simulink model "SA_50_SIMPLE_MOSFET"  (R2021a)
settings: Solver=VariableStepAuto  StartTime=0.0  StopTime=simTime  RelTol=1e-3
undefined symbols (not defined in the file or in its folder): Iend, Inom, Ion, linearMPC, Lithium, modelSelection, nomAirP, nomFuelP, nomH20comp, nomH2comp, nomO2comp, powerProfile, sigbuilder_block, slow_linearMPC, v_0A, v_1A, Vend, Vnom
libraries: spsCurrentMeasurementLib x3, spsControlledCurrentSourceLib x2, spspowerguiLib x1, spsBatteryLib x1, spsControlledVoltageSourceLib x1, spsDiodeLib x1, spsFirstOrderFilterLib x1, spsFuelCellStackLib x1, spsSeriesRLCBranchLib x1
settings Model: Creator=leonardopalacios  LastModifiedBy=leonardopalacios
settings SolverCC: ZeroCrossAlgorithm=Adaptive
settings DebuggingCC: MaskedZcDiagnostic=none  IgnoredZcDiagnostic=none

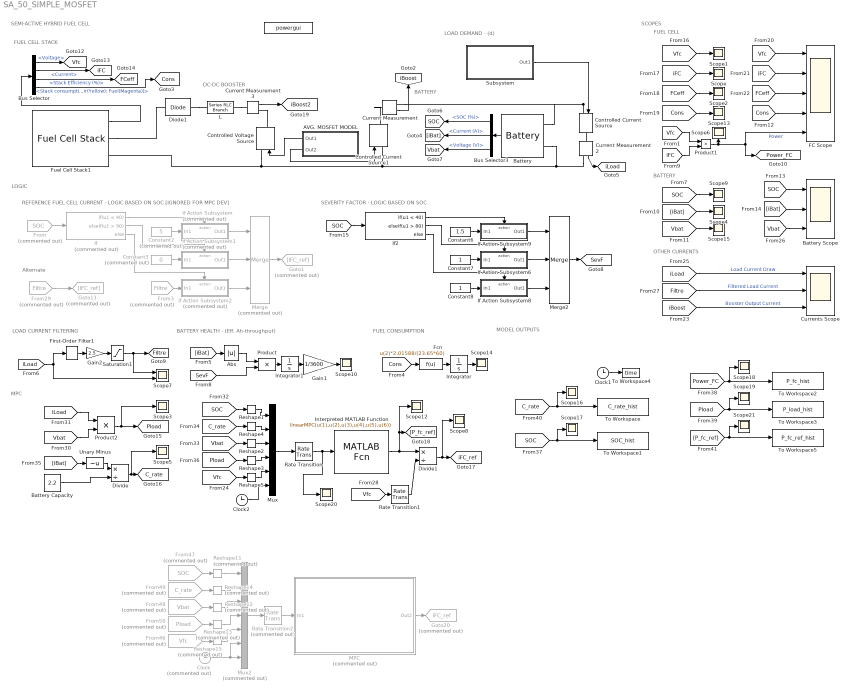
== system SA_50_SIMPLE_MOSFET ==
  note: MODEL OUTPUTS
  note: REFERENCE FUEL CELL CURRENT - LOGIC BASED ON SOC [IGNORED FOR MPC DEV]
  note: BATTERY HEALTH - (Eff. Ah-throughput)
  note: FUEL CELL STACK
  note: LOAD DEMAND - (d)
  note: OTHER CURRENTS
  note: FUEL CONSUMPTION
  note: LOGIC
  note: DC-DC BOOSTER
  note: SEVERITY FACTOR - LOGIC BASED ON SOC
  note: FUEL CELL
  note: BATTERY
  note: BATTERY
  note: LOAD CURRENT FILTERING
  note: SEMI-ACTIVE HYBRID FUEL CELL
  note: SCOPES
  note: MPC
  note: Alternate
  " " : spspowerguiLib/powergui  Priority=1  SimulationMode=Continuous  SampleTime=50e-6  frequency=60  Iterations=50  frequencyindice=0  Pbase=100e6  ErrMax=1e-4  UnitsV=kV  UnitsW=MW  buscounter=0  FunctionMessages=off  echomessages=off  EnableUseOfTLC=off  CurrentSourceSwitches=off  DisableSnubberDevices=off  DisableRonSwitches=off  DisableVfSwitches=off  DisplayEquations=off  AutomaticDiscreteSolvers=off  SolverType=Tustin/Backward Euler (TBE)  Interpol=off  ExternalGateDelay=off  methode=off  Ts=10  x0status=blocks  SPID=off  SwTol=0  HookPort=off  NonlinearTolerance=1e-4  nMaxIteration=100  ContinueOnMaxIteration=off  RestoreLinks=warning  ResistiveCurrentMeasurement=off  Frange=[0:2:500]  Ylog=off  Xlog=on  ShowGrid=off  save=off  variable=ZData  structure=0  ZoomFFT=off  StartTime=0.0  cycles=1  DisplayStyle=1  fundamental=60  FreqAxis=off  MaxFrequency=1000  frequencyindicesteady=1  RmsSteady=1  display=off
  AVG. MOSFET MODEL : Subsystem
  Abs : Abs
  Battery : spsBatteryLib/Battery  BatType=Lithium-Ion  ShowTempParam=off  ThermalPreset=no  ShowAgeParam=off  NomV=bat_nom_V  NomQ=capacity  SOC=SoC_init  Batt_Tr=bat_tau  PresetModel=on  MaxQ=2.2  MinV=30  FullV=46.5595  Dis_rate=0.95652  R=0.18182  Normal_OP=1.9896  expZone="[43.2154     0.108087]"  current=[6.5 13 32.5]  Units=Time  Tci=20  NomT=25  T2=0  MaxQ2=2.208  FullV2=3.45  Normal_OP2=2.8  expZone2="[3.22        0.23]"  Rca=0.6  ti=1000  Dp=0  Neq0=0  Tsim=1e6  Ta1=25  Qeol=5.4*0.9  Reol=0.013333*1.2  Char_age=[2.3478, 3]  Dis_age=[2.3478, 10]  N1=1500  N2=10500  N3=1000  N4=1400  Ta2=45  N5=950
  Battery Capacity : Constant  Value=2.2
  "Battery Scope " : Scope  NumInputPorts=3
  Bus Selector : BusSelector  OutputSignals=Voltage,Current,Stack Efficiency (%),Stack consumption (Standard lpm) [Air(Yellow); Fuel(Magenta)]
  Bus Selector3 : BusSelector  OutputSignals=SOC (%),Current (A),Voltage (V)
  Clock : Clock  Commented=on
  Clock1 : Clock
  Clock2 : Clock
  Constant2 : Constant  Commented=on  Value=5
  Constant3 : Constant  Commented=on  Value=0
  Constant6 : Constant  Value=1.5
  Constant7 : Constant
  Constant8 : Constant
  Controlled Current Source : spsControlledCurrentSourceLib/Controlled Current Source  Initialize=off  Source_Type=DC  Amplitude=0  Phase=0  Frequency=0  Measurements=Current
  Controlled Current Source1 : spsControlledCurrentSourceLib/Controlled Current Source  Initialize=on  Source_Type=DC  Amplitude=0  Phase=0  Frequency=0  Measurements=Current
  Controlled Voltage Source : spsControlledVoltageSourceLib/Controlled Voltage Source  Initialize=on  Source_Type=DC  Amplitude=32.5  Phase=0  Frequency=0  Measurements=None
  Current Measurement : spsCurrentMeasurementLib/Current Measurement  PhasorSimulation=off  OutputType=Complex  PSBequivalent=0
  Current Measurement2 : spsCurrentMeasurementLib/Current Measurement  PhasorSimulation=off  OutputType=Complex  PSBequivalent=0
  Current Measurement3 : spsCurrentMeasurementLib/Current Measurement  PhasorSimulation=off  OutputType=Complex  PSBequivalent=0
  "Currents Scope " : Scope  NumInputPorts=3
  Diode1 : spsDiodeLib/Diode  Ron=0.001  Lon=0  Vf=0.8  IC=0  UseSnubber=off  Rs=500  Cs=250e-9  Measurements=off
  Divide : Product  Inputs=*/
  Divide1 : Product  Inputs=*/
  FC Scope : Scope  NumInputPorts=5
  Fcn : Fcn  Expr=u(2)*2.01588/(23.65*60)
  First-Order Filter1 : spsFirstOrderFilterLib/First-Order Filter  FilterType=Lowpass  Tc=5  Ts=0  Initialize=on  Vac_Init=[0, 0, 60]  Vdc_Init=1.1  PlotResponse=off  FreqRange="[0,  200,  1]"
  From : From  Commented=on  GotoTag=SOC
  From29 : From  Commented=on  GotoTag=Filtre
  From3 : From  Commented=on  GotoTag=Filtre
  From46 : From  Commented=on  GotoTag=Vfc  TagVisibility=global
  From47 : From  Commented=on  GotoTag=SOC  TagVisibility=global
  From48 : From  Commented=on  GotoTag=Vbat  TagVisibility=global
  From49 : From  Commented=on  GotoTag=C_rate  TagVisibility=global
  From50 : From  Commented=on  GotoTag=Pload  TagVisibility=global
  Fuel Cell Stack1 : spsFuelCellStackLib/Fuel Cell Stack  PresetModel=No (User-Defined)  FcType=0  Detailed=Detailed  Eoc=[v_0A, v_1A]  NomVI=[Inom, Vnom]  EndVI=[Iend, Vend]  Nc=nCells  n=stackEff  TOp=opTemp  AirFr=nomAir  SuppPress=[nomFuelP, nomAirP]  Comp=[nomH2comp, nomO2comp, nomH20comp]  SignX=off  SignY=off  FlowRateH2=off  FlowRateAir=off  SystemTemp=off  SystemPH2=off  SystemPAir=off  FCDyn=off  FC_tau=1  Peak_O2=80  V_Under=10
      settings: SourceProductBaseCode=PS
  Gain1 : Gain  Gain=1/3600
  Gain2 : Gain  Gain=2.5
  Goto1 : Goto  Commented=on  GotoTag=iFC_ref
  Goto11 : Goto  Commented=on  GotoTag=iFC_ref
  Goto20 : Goto  Commented=on  GotoTag=iFC_ref  TagVisibility=global
  If : If  Commented=on  IfExpression=u1 < 40  ElseIfExpressions=u1 > 90
  If Action Subsystem : Subsystem  Commented=on  TreatAsAtomicUnit=on
  If Action Subsystem1 : Subsystem  Commented=on  TreatAsAtomicUnit=on
  If Action Subsystem2 : Subsystem  Commented=on  TreatAsAtomicUnit=on
  If Action Subsystem6 : Subsystem  TreatAsAtomicUnit=on
  If Action Subsystem8 : Subsystem  TreatAsAtomicUnit=on
  If Action Subsystem9 : Subsystem  TreatAsAtomicUnit=on
  If2 : If  IfExpression=u1 < 40  ElseIfExpressions=u1 > 80
  Integrator : Integrator
  Integrator1 : Integrator
  Interpreted MATLAB Function : MATLABFcn  MATLABFcn=linearMPC(u(1),u(2),u(3),u(4),u(5),u(6))
  L : spsSeriesRLCBranchLib/Series RLC Branch  LConnTagsString=__new0  RConnTagsString=__new0  BranchType=L  Resistance=1  Inductance=100e-3  SetiL0=off  InitialCurrent=0  Capacitance=1e-6  Setx0=off  InitialVoltage=0  Measurements=None
  MPC : Subsystem  Commented=on
  Merge : Merge  Commented=on  Inputs=3
  Merge2 : Merge  Inputs=3
  Mux : Mux  Inputs=6
  Mux2 : Mux  Commented=on  Inputs=7
  Product : Product
  Product1 : Product
  Product2 : Product
  Rate Transition : RateTransition  OutPortSampleTime=Ts
  Rate Transition1 : RateTransition  OutPortSampleTime=Ts
  Rate Transition2 : RateTransition  Commented=on  OutPortSampleTime=Ts
  Reshape{1..5} (5 alike) : Reshape  OutputDimensionality=Customize  OutputDimensions=1
  Reshape{11..15} (5 alike) : Reshape  Commented=on  OutputDimensionality=Customize  OutputDimensions=1
  Saturation1 : Saturate  UpperLimit=5  LowerLimit=0
  Scope{,1..6,8..10,12..21} (20 alike) : Scope
  Scope7 : Scope  NumInputPorts=2
  Subsystem : Subsystem
  To Workspace : ToWorkspace  VariableName=C_rate_hist  SaveFormat=Timeseries  SampleTime=-1
  To Workspace1 : ToWorkspace  VariableName=SOC_hist  SaveFormat=Timeseries  SampleTime=-1
  To Workspace2 : ToWorkspace  VariableName=P_fc_hist  SaveFormat=Timeseries  SampleTime=-1
  To Workspace3 : ToWorkspace  VariableName=P_load_hist  SaveFormat=Timeseries  SampleTime=-1
  To Workspace4 : ToWorkspace  VariableName=time  SaveFormat=Timeseries  SampleTime=-1
  To Workspace5 : ToWorkspace  VariableName=P_fc_ref_hist  SaveFormat=Timeseries  SampleTime=-1
  Unary Minus : UnaryMinus
  tag scope: C_rate=global, Cons=global, FCeff=global, Filtre=global, Pload=global, Power_FC=global, SOC=global, SevF=global, Vbat=global, Vfc=global, iBoost2=global, iBoost=global, iFC=global, iFC_ref=global, iLoad=global
  wires:
  Battery/1 -> Bus Selector3/1
  [SevF] -> Product/2
  Product/1 -> Integrator1/1
  [Vfc] -> FC Scope/1
  [Vfc] -> Product1/1
  [iBat] -> Unary Minus/1
  Current Measurement2/1 -> [iLoad]
  [Vbat] -> Reshape2/1
  Reshape2/1 -> Mux/3
  First-Order Filter1/1 -> Gain2/1
  Product1/1 -> FC Scope/5, [Power_FC], Scope6/1  "Power"
  [iLoad] -> Product2/1
  [Pload] -> Scope19/1, To Workspace3/1
  Constant3/1 -> If Action Subsystem1/1(In1)
  [FCeff] -> FC Scope/3
  Reshape4/1 -> Mux/2
  [Vbat] -> "Battery Scope "/3
  Clock1/1 -> To Workspace4/1
  Bus Selector/1 -> [Vfc]  "<Voltage>"
  [P_fc_ref] -> Scope21/1, To Workspace5/1
  Reshape3/1 -> Mux/4
  Reshape5/1 -> Mux/5
  Bus Selector/2 -> [iFC]  "<Current>"
  Current Measurement/1 -> [iBoost]
  Mux/1 -> Rate Transition/1
  Gain2/1 -> Saturation1/1
  [SOC] -> Scope17/1, To Workspace1/1
  Bus Selector3/3 -> [Vbat]  "<Voltage (V)>"
  [Cons] -> Fcn/1
  If Action Subsystem9/1(Out1) -> Merge2/1
  If Action Subsystem2/1(Out1) -> Merge/3
  Constant8/1 -> If Action Subsystem8/1(In1)
  If/1 -> If Action Subsystem/Action
  Rate Transition1/1 -> Divide1/2
  If2/2 -> If Action Subsystem6/Action
  If/2 -> If Action Subsystem1/Action
  Integrator/1 -> Scope14/1
  Fcn/1 -> Integrator/1
  Bus Selector/4 -> [Cons]  "<Stack consumption (Standard lpm) [Air(Yellow); Fuel(Magenta)]>"
  [SOC] -> Reshape1/1
  If Action Subsystem/1(Out1) -> Merge/1
  Fuel Cell Stack1/1 -> Bus Selector/1
  Battery Capacity/1 -> Divide/2
  [iBat] -> Abs/1
  Bus Selector/3 -> [FCeff]  "<Stack Efficiency (%)>"
  [iBat] -> "Battery Scope "/2
  [iBoost] -> "Currents Scope "/3  "Booster Output Current"
  Abs/1 -> Product/1
  Merge/1 -> Goto1/1
  From29/1 -> Goto11/1
  [Cons] -> FC Scope/4
  If/3 -> If Action Subsystem2/Action
  Divide/1 -> Scope5/1, [C_rate]
  Saturation1/1 -> [Filtre], Scope7/1
  [iLoad] -> "Currents Scope "/1  "Load Current Draw"
  Bus Selector3/1 -> [SOC]  "<SOC (%)>"
  Constant2/1 -> If Action Subsystem/1(In1)
  [C_rate] -> Reshape4/1
  [Filtre] -> "Currents Scope "/2  "Filtered Load Current"
  Divide1/1 -> Scope8/1, [iFC_ref]
  [Vbat] -> Product2/2
  From/1 -> If/1
  Product2/1 -> Scope3/1, [Pload]
  [Power_FC] -> To Workspace2/1, Scope18/1
  [FCeff] -> Scope2/1
  [SOC] -> "Battery Scope "/1
  If Action Subsystem8/1(Out1) -> Merge2/3
  Bus Selector3/2 -> [iBat]  "<Current (A)>"
  [iFC] -> FC Scope/2
  Reshape1/1 -> Mux/1
  [Pload] -> Reshape3/1
  If2/1 -> If Action Subsystem9/Action
  Constant6/1 -> If Action Subsystem9/1(In1)
  [SOC] -> Scope9/1
  [Vfc] -> Reshape5/1
  [iFC] -> Scope/1
  Constant7/1 -> If Action Subsystem6/1(In1)
  Rate Transition/1 -> Scope20/1, Interpreted MATLAB Function/1
  Unary Minus/1 -> Divide/1
  [C_rate] -> To Workspace/1, Scope16/1
  Merge2/1 -> [SevF]
  [Vfc] -> Rate Transition1/1
  Interpreted MATLAB Function/1 -> [P_fc_ref], Scope12/1, Divide1/1
  [iLoad] -> Scope7/2, First-Order Filter1/1
  [Vbat] -> Scope15/1
  [Vfc] -> Scope1/1
  [iBat] -> Scope4/1
  [Cons] -> Scope13/1
  Integrator1/1 -> Gain1/1
  Gain1/1 -> Scope10/1
  [iFC] -> Product1/2
  If Action Subsystem1/1(Out1) -> Merge/2
  If2/3 -> If Action Subsystem8/Action
  [SOC] -> If2/1
  From3/1 -> If Action Subsystem2/1(In1)
  If Action Subsystem6/1(Out1) -> Merge2/2
  Current Measurement3/1 -> [iBoost2]
  AVG. MOSFET MODEL/2(Out2) -> Controlled Current Source1/1
  AVG. MOSFET MODEL/1(Out1) -> Controlled Voltage Source/1
  Subsystem/1(Out1) -> Controlled Current Source/1
  Rate Transition2/1 -> MPC/1(In1)
  MPC/1(Out2) -> Goto20/1
  From46/1 -> Reshape15/1
  Reshape14/1 -> Mux2/2
  From49/1 -> Reshape14/1
  Reshape11/1 -> Mux2/1
  Reshape12/1 -> Mux2/3
  From50/1 -> Reshape13/1
  From47/1 -> Reshape11/1
  Reshape13/1 -> Mux2/4
  From48/1 -> Reshape12/1
  Reshape15/1 -> Mux2/5
  Mux2/1 -> Rate Transition2/1
  Clock/1 -> Mux2/7, Mux2/6
  Clock2/1 -> Mux/6
  connections:
  Controlled Current Source/LConn1 -- Current Measurement/RConn1 -- Battery/LConn1
  Battery/LConn2 -- Current Measurement2/RConn1 -- Controlled Voltage Source/LConn1 -- Fuel Cell Stack1/RConn2 -- Controlled Current Source1/LConn1
  Current Measurement3/RConn1 -- Controlled Voltage Source/RConn1
  Current Measurement/LConn1 -- Controlled Current Source1/RConn1
  Controlled Current Source/RConn1 -- Current Measurement2/LConn1
  L/RConn1 -- Current Measurement3/LConn1
  Fuel Cell Stack1/RConn1 -- Diode1/LConn1
  Diode1/RConn1 -- L/LConn1

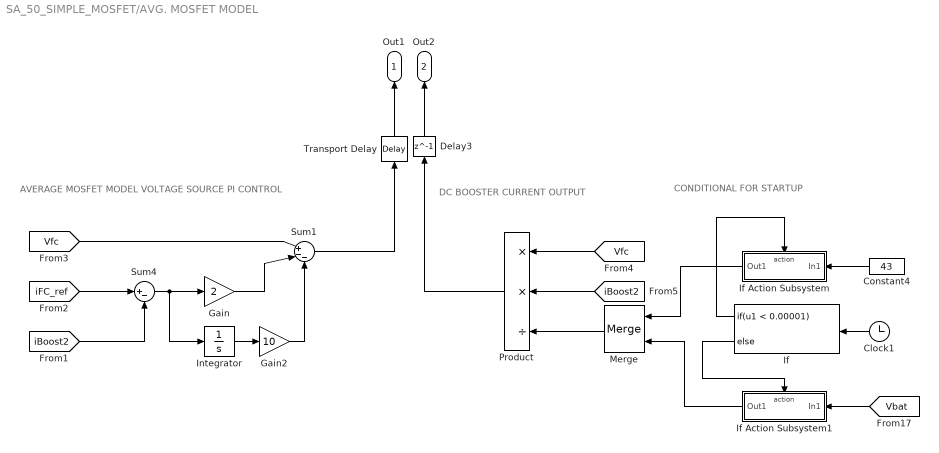
== system SA_50_SIMPLE_MOSFET/AVG. MOSFET MODEL ==
  note: AVERAGE MOSFET MODEL VOLTAGE SOURCE PI CONTROL
  note: DC BOOSTER CURRENT OUTPUT
  note: CONDITIONAL FOR STARTUP
  Clock1 : Clock
  Constant4 : Constant  Value=43
  Delay3 : Delay  DelayLength=1
  Gain : Gain  Gain=2
  Gain2 : Gain  Gain=10
  If : If  IfExpression=u1 < 0.00001
  If Action Subsystem : Subsystem  TreatAsAtomicUnit=on
  If Action Subsystem1 : Subsystem  TreatAsAtomicUnit=on
  Integrator : Integrator
  Merge : Merge
  Product : Product  Inputs=**/
  Sum1 : Sum  Inputs=|+--
  Sum4 : Sum  Inputs=|+-
  Transport Delay : TransportDelay  DelayTime=0.00000000001
  Out1 : Outport
  Out2 : Outport  Port=2
  wires:
  [Vbat] -> If Action Subsystem1/1(In1)
  Product/1 -> Delay3/1
  [Vfc] -> Sum1/1
  Gain/1 -> Sum1/2
  If/1 -> If Action Subsystem/Action
  [iBoost2] -> Sum4/2
  If/2 -> If Action Subsystem1/Action
  Sum4/1 -> Integrator/1, Gain/1
  Merge/1 -> Product/3
  Constant4/1 -> If Action Subsystem/1(In1)
  Integrator/1 -> Gain2/1
  Clock1/1 -> If/1
  Gain2/1 -> Sum1/3
  [iFC_ref] -> Sum4/1
  If Action Subsystem/1(Out1) -> Merge/1
  If Action Subsystem1/1(Out1) -> Merge/2
  Delay3/1 -> Out2/1
  [iBoost2] -> Product/2
  [Vfc] -> Product/1
  Sum1/1 -> Transport Delay/1
  Transport Delay/1 -> Out1/1

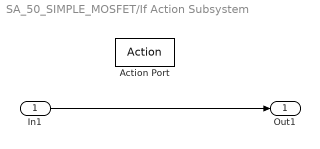
== system SA_50_SIMPLE_MOSFET/If Action Subsystem ==
  In1 : Inport
  Action Port : ActionPort  ActionPortLabel=if(u1 < 40)
  Out1 : Outport
  wires:
  In1/1 -> Out1/1

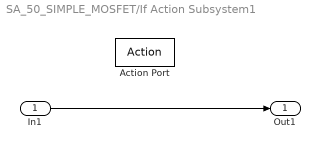
== system SA_50_SIMPLE_MOSFET/If Action Subsystem1 ==
  In1 : Inport
  Action Port : ActionPort  ActionPortLabel=elseif(u1 > 90)
  Out1 : Outport
  wires:
  In1/1 -> Out1/1

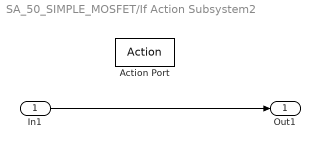
== system SA_50_SIMPLE_MOSFET/If Action Subsystem2 ==
  In1 : Inport
  Action Port : ActionPort  ActionPortLabel=else
  Out1 : Outport
  wires:
  In1/1 -> Out1/1

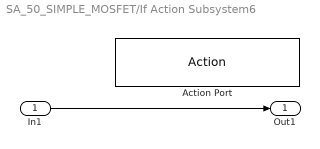
== system SA_50_SIMPLE_MOSFET/If Action Subsystem6 ==
  In1 : Inport
  Action Port : ActionPort  ActionPortLabel=elseif(u1 > 80)
  Out1 : Outport
  wires:
  In1/1 -> Out1/1

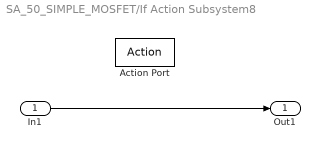
== system SA_50_SIMPLE_MOSFET/If Action Subsystem8 ==
  In1 : Inport
  Action Port : ActionPort  ActionPortLabel=else
  Out1 : Outport
  wires:
  In1/1 -> Out1/1

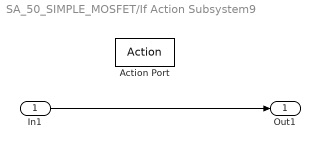
== system SA_50_SIMPLE_MOSFET/If Action Subsystem9 ==
  In1 : Inport
  Action Port : ActionPort  ActionPortLabel=if(u1 < 40)
  Out1 : Outport
  wires:
  In1/1 -> Out1/1

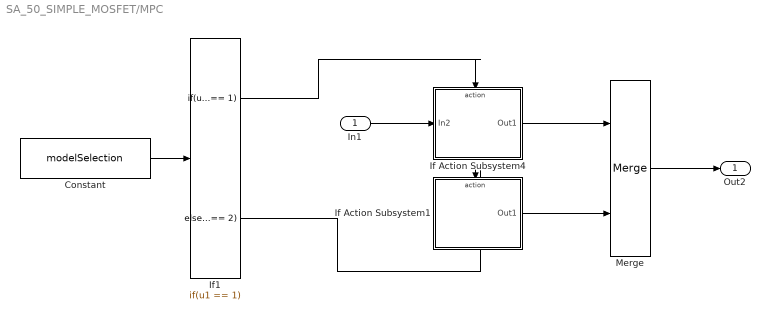
== system SA_50_SIMPLE_MOSFET/MPC ==
  In1 : Inport
  Constant : Constant  Value=modelSelection
  If Action Subsystem1 : Subsystem  TreatAsAtomicUnit=on
  If Action Subsystem4 : Subsystem  TreatAsAtomicUnit=on
  If1 : If  IfExpression=u1 == 1  ElseIfExpressions=u1 == 2  ShowElse=off
  Merge : Merge
  Out2 : Outport
  wires:
  If1/1 -> If Action Subsystem4/Action
  Constant/1 -> If1/1
  If1/2 -> If Action Subsystem1/Action
  In1/1 -> If Action Subsystem4/1(In2)
  If Action Subsystem1/1(Out1) -> Merge/2
  If Action Subsystem4/1(Out1) -> Merge/1
  Merge/1 -> Out2/1

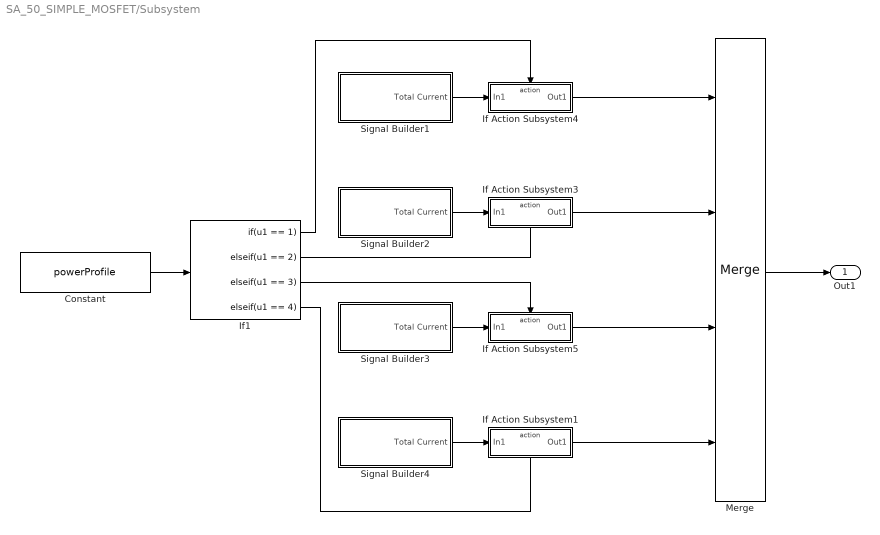
== system SA_50_SIMPLE_MOSFET/Subsystem ==
  Constant : Constant  Value=powerProfile
  If Action Subsystem1 : Subsystem  TreatAsAtomicUnit=on
  If Action Subsystem3 : Subsystem  TreatAsAtomicUnit=on
  If Action Subsystem4 : Subsystem  TreatAsAtomicUnit=on
  If Action Subsystem5 : Subsystem  TreatAsAtomicUnit=on
  If1 : If  IfExpression=u1 == 1  ElseIfExpressions=u1 == 2, u1 == 3, u1 == 4  ShowElse=off
  Merge : Merge  Inputs=4
  Signal Builder1 : Subsystem  Tag=STV Subsys  LoadFcn=sigbuilder_block('load');  StartFcn=sigbuilder_block('start');  StopFcn=sigbuilder_block('stop');  ClipboardFcn=sigbuilder_block('clipboard');  mask(Sigbuilder block){tuvar=[0:10]}
      mask help: Simulink:masks:SigbuilderBlock_MD
      mask init:
      | if ~strcmp(get_param(bdroot(gcbh),'SimulationStatus'),'stopped') tuvar = sigbuilder_block('maskInit'); end
      settings: CopyFcn=sigbuilder_block('copy');  DeleteFcn=sigbuilder_block('delete');  ModelCloseFcn=sigbuilder_block('modelClose');  PreSaveFcn=sigbuilder_block('preSave');  PauseFcn=sigbuilder_block('pause');  ContinueFcn=sigbuilder_block('continue');  NameChangeFcn=sigbuilder_block('namechange');  OpenFcn=sigbuilder_block('open',[73 196 1706 550 ]);  CloseFcn=sigbuilder_block('close');
      mask Display: plot(0, 0, 100, 100,[2, 2, 32, 32, 2], [68, 8, 8, 68, 68],[32, 2], [38, 38], [32, 19, 2],[53, 60, 44], [32, 17, 17, 2],[16, 16, 31, 31]);txt = getActiveGroup(gcbh);text(2, 100, txt,'verticalAlignment', 'top');
  Signal Builder2 : Subsystem  Tag=STV Subsys  LoadFcn=sigbuilder_block('load');  StartFcn=sigbuilder_block('start');  StopFcn=sigbuilder_block('stop');  ClipboardFcn=sigbuilder_block('clipboard');  mask(Sigbuilder block){tuvar=[0:10]}
      mask help: Simulink:masks:SigbuilderBlock_MD
      mask init:
      | if ~strcmp(get_param(bdroot(gcbh),'SimulationStatus'),'stopped') tuvar = sigbuilder_block('maskInit'); end
      settings: CopyFcn=sigbuilder_block('copy');  DeleteFcn=sigbuilder_block('delete');  ModelCloseFcn=sigbuilder_block('modelClose');  PreSaveFcn=sigbuilder_block('preSave');  PauseFcn=sigbuilder_block('pause');  ContinueFcn=sigbuilder_block('continue');  NameChangeFcn=sigbuilder_block('namechange');  OpenFcn=sigbuilder_block('open',[73 196 1706 550 ]);  CloseFcn=sigbuilder_block('close');
      mask Display: plot(0, 0, 100, 100,[2, 2, 32, 32, 2], [68, 8, 8, 68, 68],[32, 2], [38, 38], [32, 19, 2],[53, 60, 44], [32, 17, 17, 2],[16, 16, 31, 31]);txt = getActiveGroup(gcbh);text(2, 100, txt,'verticalAlignment', 'top');
  Signal Builder3 : Subsystem  Tag=STV Subsys  LoadFcn=sigbuilder_block('load');  StartFcn=sigbuilder_block('start');  StopFcn=sigbuilder_block('stop');  ClipboardFcn=sigbuilder_block('clipboard');  mask(Sigbuilder block){tuvar=[0:10]}
      mask help: Simulink:masks:SigbuilderBlock_MD
      mask init:
      | if ~strcmp(get_param(bdroot(gcbh),'SimulationStatus'),'stopped') tuvar = sigbuilder_block('maskInit'); end
      settings: CopyFcn=sigbuilder_block('copy');  DeleteFcn=sigbuilder_block('delete');  ModelCloseFcn=sigbuilder_block('modelClose');  PreSaveFcn=sigbuilder_block('preSave');  PauseFcn=sigbuilder_block('pause');  ContinueFcn=sigbuilder_block('continue');  NameChangeFcn=sigbuilder_block('namechange');  OpenFcn=sigbuilder_block('open',[73 196 1706 550 ]);  CloseFcn=sigbuilder_block('close');
      mask Display: plot(0, 0, 100, 100,[2, 2, 32, 32, 2], [68, 8, 8, 68, 68],[32, 2], [38, 38], [32, 19, 2],[53, 60, 44], [32, 17, 17, 2],[16, 16, 31, 31]);txt = getActiveGroup(gcbh);text(2, 100, txt,'verticalAlignment', 'top');
  Signal Builder4 : Subsystem  Tag=STV Subsys  LoadFcn=sigbuilder_block('load');  StartFcn=sigbuilder_block('start');  StopFcn=sigbuilder_block('stop');  ClipboardFcn=sigbuilder_block('clipboard');  mask(Sigbuilder block){tuvar=[0:10]}
      mask help: Simulink:masks:SigbuilderBlock_MD
      mask init:
      | if ~strcmp(get_param(bdroot(gcbh),'SimulationStatus'),'stopped') tuvar = sigbuilder_block('maskInit'); end
      settings: CopyFcn=sigbuilder_block('copy');  DeleteFcn=sigbuilder_block('delete');  ModelCloseFcn=sigbuilder_block('modelClose');  PreSaveFcn=sigbuilder_block('preSave');  PauseFcn=sigbuilder_block('pause');  ContinueFcn=sigbuilder_block('continue');  NameChangeFcn=sigbuilder_block('namechange');  OpenFcn=sigbuilder_block('open',[73 196 1706 550 ]);  CloseFcn=sigbuilder_block('close');
      mask Display: plot(0, 0, 100, 100,[2, 2, 32, 32, 2], [68, 8, 8, 68, 68],[32, 2], [38, 38], [32, 19, 2],[53, 60, 44], [32, 17, 17, 2],[16, 16, 31, 31]);txt = getActiveGroup(gcbh);text(2, 100, txt,'verticalAlignment', 'top');
  Out1 : Outport
  wires:
  Merge/1 -> Out1/1
  If1/1 -> If Action Subsystem4/Action
  Constant/1 -> If1/1
  If1/4 -> If Action Subsystem1/Action
  If Action Subsystem3/1(Out1) -> Merge/2
  If Action Subsystem5/1(Out1) -> Merge/3
  Signal Builder3/1(Total Current) -> If Action Subsystem5/1(In1)
  If1/2 -> If Action Subsystem3/Action
  Signal Builder1/1(Total Current) -> If Action Subsystem4/1(In1)
  Signal Builder4/1(Total Current) -> If Action Subsystem1/1(In1)
  If Action Subsystem1/1(Out1) -> Merge/4
  Signal Builder2/1(Total Current) -> If Action Subsystem3/1(In1)
  If Action Subsystem4/1(Out1) -> Merge/1
  If1/3 -> If Action Subsystem5/Action

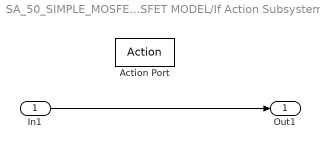
== system SA_50_SIMPLE_MOSFET/AVG. MOSFET MODEL/If Action Subsystem ==
  In1 : Inport
  Action Port : ActionPort  ActionPortLabel=if(u1 < 0.00001)
  Out1 : Outport
  wires:
  In1/1 -> Out1/1

== system SA_50_SIMPLE_MOSFET/AVG. MOSFET MODEL/If Action Subsystem1 ==
  In1 : Inport
  Action Port : ActionPort  ActionPortLabel=else
  Out1 : Outport
  wires:
  In1/1 -> Out1/1

== system SA_50_SIMPLE_MOSFET/MPC/If Action Subsystem1 ==
  Action Port : ActionPort  ActionPortLabel=elseif(u1 == 2)
  Constant : Constant  Value=0
  Out1 : Outport
  wires:
  Constant/1 -> Out1/1

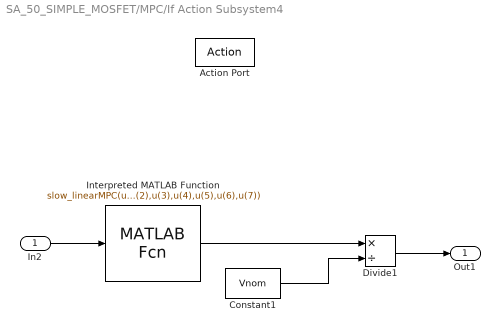
== system SA_50_SIMPLE_MOSFET/MPC/If Action Subsystem4 ==
  In2 : Inport
  Action Port : ActionPort  ActionPortLabel=if(u1 == 1)
  Constant1 : Constant  Value=Vnom
  Divide1 : Product  Inputs=*/
  Interpreted MATLAB Function : MATLABFcn  MATLABFcn=slow_linearMPC(u(1),u(2),u(3),u(4),u(5),u(6),u(7))
  Out1 : Outport
  wires:
  Constant1/1 -> Divide1/2
  Interpreted MATLAB Function/1 -> Divide1/1
  Divide1/1 -> Out1/1
  In2/1 -> Interpreted MATLAB Function/1

== system SA_50_SIMPLE_MOSFET/Subsystem/If Action Subsystem1 ==
  In1 : Inport
  Action Port : ActionPort  ActionPortLabel=elseif( u1 == 4 )
  Out1 : Outport
  wires:
  In1/1 -> Out1/1

== system SA_50_SIMPLE_MOSFET/Subsystem/If Action Subsystem3 ==
  In1 : Inport
  Action Port : ActionPort  ActionPortLabel=elseif(u1 == 2)
  Out1 : Outport
  wires:
  In1/1 -> Out1/1

== system SA_50_SIMPLE_MOSFET/Subsystem/If Action Subsystem4 ==
  In1 : Inport
  Action Port : ActionPort  ActionPortLabel=if(u1 == 1)
  Out1 : Outport
  wires:
  In1/1 -> Out1/1

== system SA_50_SIMPLE_MOSFET/Subsystem/If Action Subsystem5 ==
  In1 : Inport
  Action Port : ActionPort  ActionPortLabel=elseif( u1 == 3)
  Out1 : Outport
  wires:
  In1/1 -> Out1/1

== system SA_50_SIMPLE_MOSFET/Subsystem/Signal Builder1 ==
  Demux : Demux  Tag=STV Demux  Outputs=1
      settings: DisplayOption=none
  FromWs : FromWorkspace  Tag=STV FromWs  VariableName=tuvar
      SigBuilderData=|
      | common.afterFinalStr = 'Extrapolate'
      | common.sampleTime = 0
      | dataSet.timeRange = [0 2048.3]
      | dataSet.name = 'Cycle1'
      | sbobj.Name = 'Signal Builder'
      | sbobj.Groups.Name = 'Cycle1'
      | sbobj.Groups.Signals.Name = 'Total Current'
      | sbobj.Groups.Signals.XData = [0 0.1 0.2 0.3 0.4 0.5 0.6 0.7 0.8 0.9 1 1.1 ... (20484 elements, 1x20484)]
      | sbobj.Groups.Signals.YData = [1.0569 1.1309 1.171 1.162 0.9589 1.143 1.056 1.261 1.1779 1.1458 1.2318 1.238 ... (20484 elements, 1x20484)]
      | sbobj.Groups.TimeRange = [0 2048.3]
  Total Current : Outport  Tag=STV Outport
  wires:
  FromWs/1 -> Demux/1
  Demux/1 -> Total Current/1

== system SA_50_SIMPLE_MOSFET/Subsystem/Signal Builder2 ==
  Demux : Demux  Tag=STV Demux  Outputs=1
      settings: DisplayOption=none
  FromWs : FromWorkspace  Tag=STV FromWs  VariableName=tuvar
      SigBuilderData=|
      | common.afterFinalStr = 'Extrapolate'
      | common.sampleTime = 0
      | dataSet.timeRange = [0 2015.9]
      | dataSet.name = 'Cycle2'
      | sbobj.Name = 'Signal Builder'
      | sbobj.Groups.Name = 'Cycle2'
      | sbobj.Groups.Signals.Name = 'Total Current'
      | sbobj.Groups.Signals.XData = [0 0.1 0.2 0.3 0.4 0.5 0.6 0.7 0.8 0.9 1 1.1 ... (20160 elements, 1x20160)]
      | sbobj.Groups.Signals.YData = [1.166 0.7379 -0.2121 1.217 1.0268 1.3439 1.34 1.221 1.1429 1.2539 0.956 1.004 ... (20160 elements, 1x20160)]
      | sbobj.Groups.TimeRange = [0 2048.3]
  Total Current : Outport  Tag=STV Outport
  wires:
  FromWs/1 -> Demux/1
  Demux/1 -> Total Current/1

== system SA_50_SIMPLE_MOSFET/Subsystem/Signal Builder3 ==
  Demux : Demux  Tag=STV Demux  Outputs=1
      settings: DisplayOption=none
  FromWs : FromWorkspace  Tag=STV FromWs  VariableName=tuvar
      SigBuilderData=|
      | common.afterFinalStr = 'Extrapolate'
      | common.sampleTime = 0
      | dataSet.timeRange = [0 2002]
      | dataSet.name = 'Cycle3'
      | sbobj.Name = 'Signal Builder'
      | sbobj.Groups.Name = 'Cycle3'
      | sbobj.Groups.Signals.Name = 'Total Current'
      | sbobj.Groups.Signals.XData = [0 0.1 0.2 0.3 0.4 0.5 0.6 0.7 0.8 0.9 1 1.1 ... (20021 elements, 1x20021)]
      | sbobj.Groups.Signals.YData = [0.003 -0.102 0.227 -0.002 0.181 0.657 0.469 0.459 1.101 1.251 0.532 1.523 ... (20021 elements, 1x20021)]
      | sbobj.Groups.TimeRange = [0 2048.3]
  Total Current : Outport  Tag=STV Outport
  wires:
  FromWs/1 -> Demux/1
  Demux/1 -> Total Current/1

== system SA_50_SIMPLE_MOSFET/Subsystem/Signal Builder4 ==
  Demux : Demux  Tag=STV Demux  Outputs=1
      settings: DisplayOption=none
  FromWs : FromWorkspace  Tag=STV FromWs  VariableName=tuvar
      SigBuilderData=|
      | common.afterFinalStr = 'Extrapolate'
      | common.sampleTime = 0
      | dataSet.timeRange = [0 2058.6]
      | dataSet.name = 'Cycle4_mod'
      | sbobj.Name = 'Signal Builder'
      | sbobj.Groups.Name = 'Cycle4_mod'
      | sbobj.Groups.Signals.Name = 'Total Current'
      | sbobj.Groups.Signals.XData = [0 0.1 0.2 0.3 0.4 0.5 0.6 0.7 0.8 0.9 1 1.1 ... (20587 elements, 1x20587)]
      | sbobj.Groups.Signals.YData = [1.081 0.135 1.5339 2.1729 1.196 1.0869 1.477 1.6258 1.0419 0.7549 0.811 0.443 ... (20587 elements, 1x20587)]
      | sbobj.Groups.TimeRange = [0 2048.3]
  Total Current : Outport  Tag=STV Outport
  wires:
  FromWs/1 -> Demux/1
  Demux/1 -> Total Current/1
